simulink model "q3_main_model"  (R2018a)
settings: Solver=VariableStepAuto  StartTime=0.0  StopTime=0.04  FixedStep=1e-6  RelTol=1e-6
libraries: powerlib x13
settings Model: Creator=burya  LastModifiedBy=burya

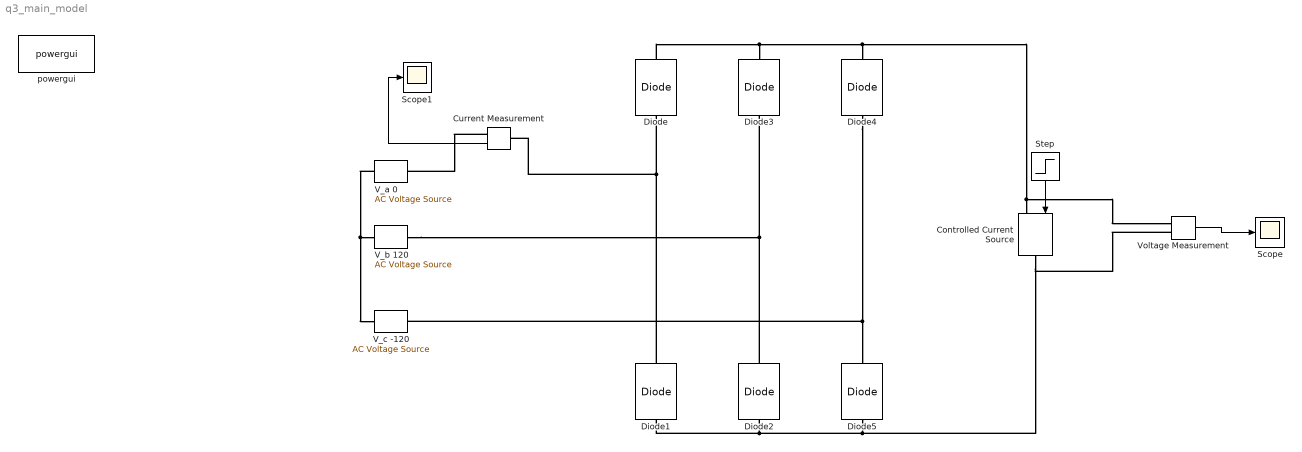
== system q3_main_model ==
  Controlled Current Source : powerlib/Electrical Sources/Controlled Current Source  Initialize=on  Source_Type=DC  Amplitude=40  Phase=0  Frequency=0  Measurements=None
  Current Measurement : powerlib/Measurements/Current Measurement  PhasorSimulation=off  OutputType=Complex  PSBequivalent=0
  Diode : powerlib/Power Electronics/Diode  Ron=1e-12  Lon=0  Vf=0  IC=0  UseSnubber=0  Rs=inf  Cs=0  Measurements=off
  Diode1 : powerlib/Power Electronics/Diode  Ron=1e-9  Lon=0  Vf=0  IC=0  UseSnubber=0  Rs=inf  Cs=0  Measurements=off
  Diode2 : powerlib/Power Electronics/Diode  Ron=1e-9  Lon=0  Vf=0  IC=0  UseSnubber=0  Rs=inf  Cs=0  Measurements=off
  Diode3 : powerlib/Power Electronics/Diode  Ron=1e-12  Lon=0  Vf=0  IC=0  UseSnubber=0  Rs=inf  Cs=0  Measurements=off
  Diode4 : powerlib/Power Electronics/Diode  Ron=1e-12  Lon=0  Vf=0  IC=0  UseSnubber=0  Rs=inf  Cs=0  Measurements=off
  Diode5 : powerlib/Power Electronics/Diode  Ron=1e-9  Lon=0  Vf=0  IC=0  UseSnubber=0  Rs=inf  Cs=0  Measurements=off
  Scope : Scope
  Scope1 : Scope
  Step : Step  Time=0  SampleTime=1e-6
  "V_a 0 " : powerlib/Electrical Sources/AC Voltage Source  Amplitude=230*sqrt(2)  Phase=0  Frequency=50  SampleTime=1e-6  Measurements=None  BusType=swing  Pref=10e3  Qref=0  Qmin=-inf  Qmax=+inf
  "V_b 120 " : powerlib/Electrical Sources/AC Voltage Source  Amplitude=230*sqrt(2)  Phase=120  Frequency=50  SampleTime=1e-6  Measurements=None  BusType=swing  Pref=10e3  Qref=0  Qmin=-inf  Qmax=+inf
  "V_c -120 " : powerlib/Electrical Sources/AC Voltage Source  Amplitude=230*sqrt(2)  Phase=-120  Frequency=50  SampleTime=1e-6  Measurements=None  BusType=swing  Pref=10e3  Qref=0  Qmin=-inf  Qmax=+inf
  Voltage Measurement : powerlib/Measurements/Voltage Measurement  PhasorSimulation=off  OutputType=Complex  PSBequivalent=0
  powergui : powerlib/powergui  Priority=1  SimulationMode=Continuous  SampleTime=1e-6  frequency=60  Iterations=50  frequencyindice=50  Pbase=100e6  ErrMax=1e-4  UnitsV=kV  UnitsW=MW  buscounter=0  FunctionMessages=off  echomessages=off  EnableUseOfTLC=off  CurrentSourceSwitches=off  DisableSnubberDevices=off  DisableRonSwitches=off  DisableVfSwitches=off  DisplayEquations=off  SolverType=Tustin/Backward Euler (TBE)  Interpol=off  ExternalGateDelay=off  methode=off  Ts=100  x0status=blocks  SPID=on  SwTol=0  HookPort=off  RestoreLinks=warning  ResistiveCurrentMeasurement=off  Frange=[0:2:500]  Ylog=off  Xlog=on  ShowGrid=off  save=off  variable=ZData  structure=output_voltage  ZoomFFT=off  StartTime=0  cycles=6  DisplayStyle=1  fundamental=300  FreqAxis=off  MaxFrequency=9000  frequencyindicesteady=1  RmsSteady=1  display=off
  wires:
  Voltage Measurement/1 -> Scope/1
  Current Measurement/1 -> Scope1/1
  Step/1 -> Controlled Current Source/1
  connections:
  Diode5/LConn1 -- Voltage Measurement/LConn2 -- Controlled Current Source/RConn1 -- Diode1/LConn1 -- Diode2/LConn1
  "V_a 0 "/LConn1 -- "V_c -120 "/LConn1 -- "V_b 120 "/LConn1
  Diode2/RConn1 -- "V_b 120 "/RConn1 -- Diode3/LConn1
  Current Measurement/RConn1 -- "V_a 0 "/RConn1
  Diode/RConn1 -- Voltage Measurement/LConn1 -- Controlled Current Source/LConn1 -- Diode4/RConn1 -- Diode3/RConn1
  Diode4/LConn1 -- "V_c -120 "/RConn1 -- Diode5/RConn1
  Diode1/RConn1 -- Current Measurement/LConn1 -- Diode/LConn1
